simulink model "testAlphaWallIn"  (R2013b)
settings: Solver=VariableStepDiscrete  StartTime=0.0  StopTime=10  RelTol=1e-3
libraries: carnot x2, simulink x1
settings Model: Creator=drhf  LastModifiedBy=drhf
settings DataIOCC: ReturnWorkspaceOutputs=on
settings OptimizationCC: InlineParams=on
settings DebuggingCC: ReadBeforeWriteMsg=DisableAll  WriteAfterWriteMsg=DisableAll  WriteAfterReadMsg=DisableAll  MultiTaskDSMMsg=none
settings ModelReferenceCC: UpdateModelReferenceTargets=IfOutOfDate
settings SFSimCC: SFSimEcho=off

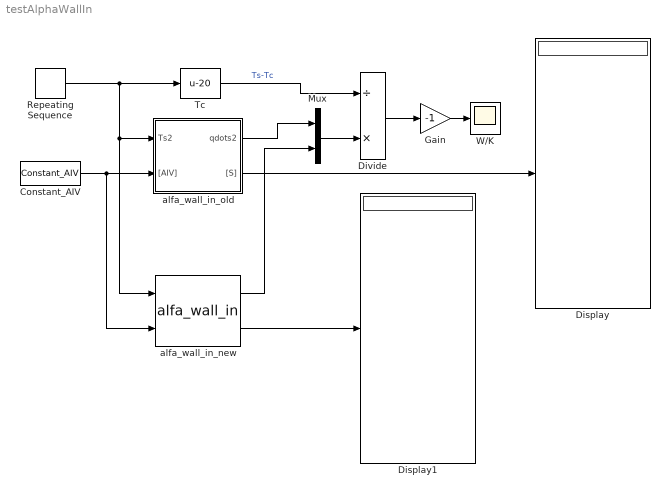
== system testAlphaWallIn ==
  Constant_AIV : carnot/Source/Ventilation/Constant_AIV  Tsens=20  Tcon=20  Trad=20  mw=0.012  mco=0.01  rhoair=1.2  cpair=1004  pair=100000  nair=0.5
  Display : Display
  Display1 : Display
  Divide : Product  Inputs=/*
  Gain : Gain  Gain=-1
  Mux : Mux  Inputs=2
  Repeating Sequence : simulink/Sources/Repeating Sequence  rep_seq_t=[0 10]  rep_seq_y=[10 30]
  Tc : Bias  Bias=-20
  W/K : Scope
  alfa_wall_in_new : carnot/Load/Houses/heat_transfer/alfa_wall_in  active=0  emission_in=0.7  wallsurface=1
  alfa_wall_in_old : Subsystem  AncestorBlock=carnot/Load/Houses/heat_transfer/alfa_wall_in  mask(ALFA){active=0, emission_in=0.7, wallsurface=1}
      mask prompts: active "Active layer (0 / 1)"; emission_in "Longwave emissivity of surface (0..1)"; wallsurface "Wall surface in m²"
      mask help:
      | Convective and radiative heat transfer at the INDOOR SURFACE of a VERTICAL OUTER WALL.
      |
      | [AIV] : conditions of zone node,
      | Ts : temperature of wall surface, °C,
      | qdots : specific heat flow into wall construction, W/m^2,
      | [S] : heat and air flow to zone node.
  wires:
  Constant_AIV/1 -> alfa_wall_in_new/2, alfa_wall_in_old/2("[AIV]")
  Repeating Sequence/1 -> alfa_wall_in_new/1, alfa_wall_in_old/1(Ts2), Tc/1
  alfa_wall_in_old/2("[S]") -> Display/1
  alfa_wall_in_new/2 -> Display1/1
  alfa_wall_in_old/1(qdots2) -> Mux/1
  alfa_wall_in_new/1 -> Mux/2
  Mux/1 -> Divide/2
  Divide/1 -> Gain/1
  Tc/1 -> Divide/1  "Ts-Tc"
  Gain/1 -> W/K/1

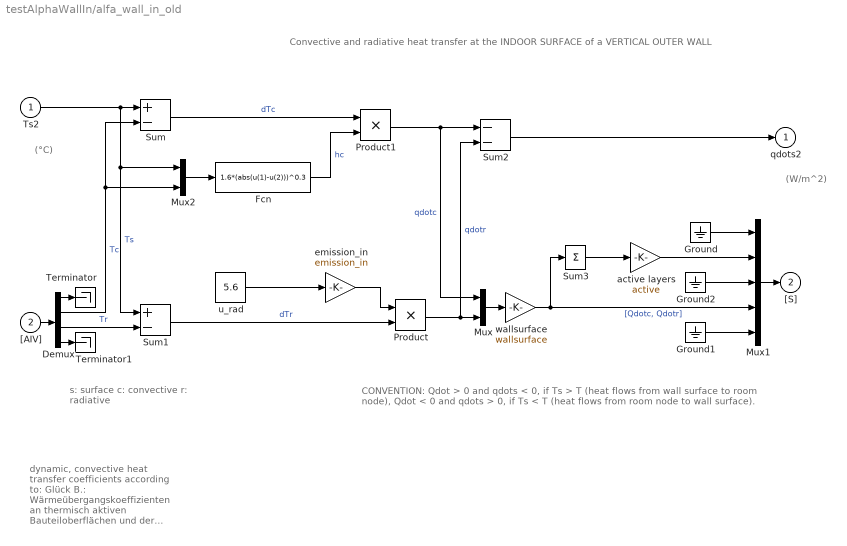
== system testAlphaWallIn/alfa_wall_in_old ==
  note: dynamic, convective heat transfer coefficients according to: Glück B.: Wärmeübergangskoeffizienten an thermisch aktiven Bauteiloberflächen
      | und der Übergang zu Basiskennlinien für die Wärmestromdichte; gi Gesundheits-Ingenieur; 128. Jahrgang 2007, Heft 1, Seiten 1-10
  note: s: surface
      | c: convective
      | r: radiative
  note: CONVENTION:
      | Qdot > 0 and qdots < 0, if Ts > T (heat flows from wall surface to room node),
      | Qdot < 0 and qdots > 0, if Ts < T (heat flows from room node to wall surface).
  note: Convective and radiative heat transfer at the INDOOR SURFACE of a VERTICAL OUTER WALL
  note: (W/m^2)
  note: (°C)
  Ts2 : Inport
  "[AIV]" : Inport  Port=2
  Demux : Demux  Outputs=[1 1 1 6]
  Fcn : Fcn  Expr=1.6*(abs(u(1)-u(2)))^0.3
  Ground : Ground
  Ground1 : Ground
  Ground2 : Ground
  Mux : Mux  Inputs=2
  Mux1 : Mux  Inputs=[4 1 1 2 5]
  Mux2 : Mux  Inputs=2
  Product : Product  SaturateOnIntegerOverflow=on  RndMeth=Zero  InputSameDT=on  OutDataTypeStr=Inherit: Same as first input
  Product1 : Product  SaturateOnIntegerOverflow=on  RndMeth=Zero  InputSameDT=on  OutDataTypeStr=Inherit: Same as first input
  Sum : Sum  Inputs=+-  SaturateOnIntegerOverflow=on  InputSameDT=on  OutDataTypeStr=Inherit: Same as first input
  Sum1 : Sum  Inputs=+-  SaturateOnIntegerOverflow=on  InputSameDT=on  OutDataTypeStr=Inherit: Same as first input
  Sum2 : Sum  Inputs=--  SaturateOnIntegerOverflow=on  InputSameDT=on  OutDataTypeStr=Inherit: Same as first input
  Sum3 : Sum  Inputs=1  SaturateOnIntegerOverflow=on  InputSameDT=on  OutDataTypeStr=Inherit: Same as first input
  Terminator : Terminator
  Terminator1 : Terminator
  active layers : Gain  Gain=active  SaturateOnIntegerOverflow=on  OutDataTypeStr=Inherit: Same as input  ParamDataTypeStr=Inherit: Same as input
  emission_in : Gain  Gain=emission_in  SaturateOnIntegerOverflow=on  OutDataTypeStr=Inherit: Same as input  ParamDataTypeStr=Inherit: Same as input
  u_rad : Constant  Value=5.6
  wallsurface : Gain  Gain=wallsurface  SaturateOnIntegerOverflow=on  OutDataTypeStr=Inherit: Same as input  ParamDataTypeStr=Inherit: Same as input
  qdots2 : Outport
  "[S]" : Outport  Port=2
  wires:
  Fcn/1 -> Product1/2  "hc"
  Product1/1 -> Mux/1, Sum2/1  "qdotc"
  Mux2/1 -> Fcn/1
  Demux/3 -> Sum1/2  "Tr"
  Sum/1 -> Product1/1  "dTc"
  Ts2/1 -> Mux2/1, Sum1/1, Sum/1  "Ts"
  u_rad/1 -> emission_in/1
  Mux/1 -> wallsurface/1
  Product/1 -> Sum2/2, Mux/2  "qdotr"
  Sum1/1 -> Product/2  "dTr"
  emission_in/1 -> Product/1
  Demux/2 -> Mux2/2, Sum/2  "Tc"
  Demux/1 -> Terminator/1
  "[AIV]"/1 -> Demux/1
  Demux/4 -> Terminator1/1
  Sum2/1 -> qdots2/1
  wallsurface/1 -> Mux1/4, Sum3/1  "[Qdotc, Qdotr]"
  Sum3/1 -> active layers/1
  Ground/1 -> Mux1/1
  Ground1/1 -> Mux1/5
  Mux1/1 -> "[S]"/1
  Ground2/1 -> Mux1/3
  active layers/1 -> Mux1/2
